simulink model "XWing"  (R2018a)
settings: Solver=VariableStepAuto  StartTime=0.0  StopTime=10.0  RelTol=1e-5  AbsTol=1e-5
PostLoadFcn:
  | Lcm = 3.2;
undefined symbols (not defined in the file): X, Y, Z
libraries: sm_lib x12, nesl_utility x4
settings Model: Creator=tdenery  LastModifiedBy=smirsky

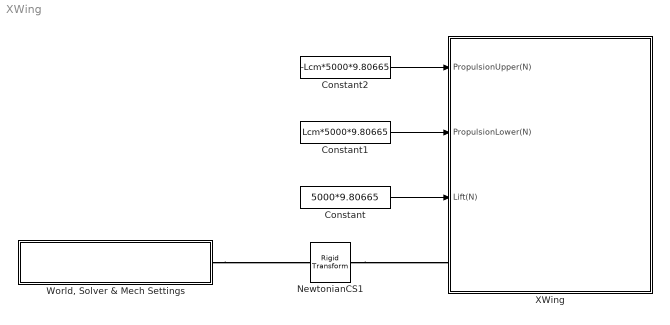
== system XWing ==
  Constant : Constant  Value=5000*9.80665
  Constant1 : Constant  Value=Lcm*5000*9.80665
  Constant2 : Constant  Value=-Lcm*5000*9.80665
  NewtonianCS1 : sm_lib/Frames and Transforms/Rigid Transform  TranslationMethod=Cartesian  TranslationStandardOffset=0  TranslationLengthUnit=m  TranslationStandardAxis=+Z  TranslationCartesianOffset=[0, 0, 0]  TranslationROffset=0  TranslationROffsetUnits=m  TranslationZOffset=0  TranslationZOffsetUnits=m  TranslationThetaOffset=0  TranslationThetaOffsetUnits=deg  RotationMethod=ArbitraryAxis  RotationAngleUnits=deg  RotationStandardAxis=+Z  RotationAngle=0  RotationArbitraryAxis=[1, 0, 0]  FollAlignAxisA=+X  BaseAlignAxisA=+Y  FollAlignAxisB=+Y  BaseAlignAxisB=+Z  RotationSequenceAxes=FollowerAxes  RotationSequence=XYX  RotationSequenceAngles=[0 0 0]  RotationSequenceAnglesUnits=deg  RotationMatrix=[1 0 0; 0 1 0; 0 0 1]
  "World, Solver & Mech Settings" : Subsystem
  XWing : Subsystem  Tag=Force/Torque  mask{PopupParam=Force/Torque}
      mask prompts: PopupParam "Motion Configuration"
      mask TypeOptions PopupParam: Force/Torque | Motion
      mask Callback PopupParam:
      | MechSystem = gcb;
      | MotionConfig = get_param( MechSystem, 'PopupParam' );
      | CurrentConfig = get_param( MechSystem, 'Tag' );
      | if ~strcmp( MotionConfig, CurrentConfig )
      |     MotOutports = find_system(MechSystem,'LookUnderMasks','all','Tag','MechSystemMotorOutport');
      |     ActOutports = find_system(MechSystem,'LookUnderMasks','all','Tag','MechSystemActuatorOutport');
      |     APOutports = find_system(MechSystem,'LookUnderMasks','all','Tag','MechSystemAPOutport');
      |     NMotors = length( MotOutports );
      |     NActuators = length( ActOutports );
      |     NActuatedPrismatics = length( APOutports );
      |     if NMotors > 0
      |         hMotOutports( NMotors ) = 0;
      |         hMotors( NMotors ) = 0;
      |         hMotInports( NMotors ) = 0;
      |         MotNameRoot{NMotors} = '';
      |     end
      |     if NActuators > 0
      |         hActOutports( NActuators ) = 0;
      |         hActuators( NActuators ) = 0;
      |         hActInports( NActuators ) = 0;
      |         ActNameRoot{NActuators} = '';
      |     end
      |     if NActuatedPrismatics > 0
      |         hAPOutports( NActuatedPrismatics ) = 0;
      |         hActuatedPrismatics( NActuatedPrismatics ) = 0;
      |         hAPInports( NActuatedPrismatics ) = 0;
      |         APNameRoot{NActuatedPrismatics} = '';
      |     end
      | 
      |     for i = 1:NMotors
      |         hMotOutports(i) = getSimulinkBlockHandle( MotOutports(i) );
      |         OutportName = get_param( hMotOutports(i), 'Name' );
      |         NameLength = length( OutportName );
      |         MotNameRoot{i} = OutportName( 1:NameLength-2 );
      |         hP = get_param( hMotOutports(i), 'PortHandles' );
      |         hL = get_param( hP.Inport, 'Line' );
      |         hMotors(i) = get_param( hL, 'SrcBlockHandle' );
      |         hpMotor(i) = get_param( hMotors(i), 'PortHandles' );
      |     end
      |     for i = 1:NActuators
      |         hActOutports(i) = getSimulinkBlockHandle( ActOutports(i) );
      |         OutportName = get_param( hActOutports(i), 'Name' );
      |         NameLength = length( OutportName );
      |         ActNameRoot{i} = OutportName( 1:NameLength-2 );
      |         hP = get_param( hActOutports(i), 'PortHandles' );
      |         hL = get_param( hP.Inport, 'Line' );
      |         hActuators(i) = get_param( hL, 'SrcBlockHandle' );
      |         hpActuator(i) = get_param( hActuators(i), 'PortHandles' );
      |     end
      |     for i = 1:NActuatedPrismatics
      |         hAPOutports(i) = getSimulinkBlockHandle( APOutports(i) );
      |         OutportName = get_param( hAPOutports(i), 'Name' );
      |         NameLength = length( OutportName );
      |         APNameRoot{i} = OutportName( 1:NameLength-2 );
      |         hP = get_param( hAPOutports(i), 'PortHandles' );
      |         hL = get_param( hP.Inport, 'Line' );
      |         hActuatedPrismatics(i) = get_param( hL, 'SrcBlockHandle' );
      |         hpActuatedPrismatic(i) = get_param( hActuatedPrismatics(i), 'PortHandles' );
      |     end
      | 
      |     if strcmp( MotionConfig, 'Force/Torque' ) || strcmp( MotionConfig, 'Motion' )
      | 
      |         for i = 1:NMotors
      |             if isempty( hpMotor(i).Inport )
      |                 hMotInports(i) = add_block( 'simulink/Sources/In1', [MechSystem, '/Fred', num2str(i)] );
      |                 OutPos = get_param( MotOutports(i), 'Position' );
      |                 InPos = OutPos{1} + [-300, 0, -300, 0];
      |                 set_param( hMotInports(i), 'Position', ['[', num2str(InPos(1)), ',', num2str(InPos(2)), ',', num2str(InPos(3)), ',', num2str(InPos(4)), ']'] );
      |                 set_param( hMotInports(i), 'Tag', 'MechSystemMotorInport' );
      |             else
      |                 hP = hpMotor(i).Inport;
      |                 hL = get_param( hP, 'Line' );
      |                 hMotInports(i) = get_param( hL, 'SrcBlockHandle' );
      |             end
      |         end
      |         for i = 1:NActuators
      |             if isempty( hpActuator(i).Inport )
      |                 hActInports(i) = add_block( 'simulink/Sources/In1', [MechSystem, '/Fred', num2str(i)] );
      |                 OutPos = get_param( ActOutports(i), 'Position' );
      |                 InPos = OutPos{1} + [-300, 0, -300, 0];
      |                 set_param( hActInports(i), 'Position', ['[', num2str(InPos(1)), ',', num2str(InPos(2)), ',', num2str(InPos(3)), ',', num2str(InPos(4)), ']'] );
      |                 set_param( hActInports(i), 'Tag', 'MechSystemACtuatorInport' );
      |             else
      |                 hP = hpActuator(i).Inport;
      |                 hL = get_param( hP, 'Line' );
      |                 hActInports(i) = get_param( hL, 'SrcBlockHandle' );
      |             end
      |         end
      |         for i = 1:NActuatedPrismatics
      |             if isempty( hpActuatedPrismatic(i).Inport )
      |                 hAPInports(i) = add_block( 'simulink/Sources/In1', [MechSystem, '/Fred', num2str(i)] );
      |                 OutPos = get_param( APOutports(i), 'Position' );
      |                 InPos = OutPos{1} + [-300, 0, -300, 0];
      |                 set_param( hAPInports(i), 'Position', ['[', num2str(InPos(1)), ',', num2str(InPos(2)), ',', num2str(InPos(3)), ',', num2str(InPos(4)), ']'] );
      |                 set_param( hAPInports(i), 'Tag', 'MechSystemACtuatorInport' );
      |             else
      |                 hP = hpActuatedPrismatic(i).Inport;
      |                 hL = get_param( hP, 'Line' );
      |                 hAPInports(i) = get_param( hL, 'SrcBlockHandle' );
      |             end
      |         end
      | 
      |         if strcmp( MotionConfig, 'Force/Torque' )
      |             set_param( MechSystem, 'Tag', 'Force/Torque' );
      |             for i = 1:NMotors
      |                 o = get_param( hMotors(i), 'Object' );
      |                 o.MotorType = 'Torque';
      |                 set_param( hMotInports(i), 'Name', [MotNameRoot{i}, '(N*m)'] );
      |                 hP = get_param( hMotInports(i), 'PortHandles' );
      |                 hL = get_param( hP.Outport, 'Line' );
      |                 if hL ~= -1
      |                     delete_line( hL );
      |                 end
      |                 add_line( MechSystem, [get_param( hMotInports(i), 'Name' ), '/1'], [get_param( hMotors(i), 'Name' ), '/1'] );
      |             end
      |             for i = 1:NActuators
      |                 o = get_param( hActuators(i), 'Object' );
      |                 o.ActuationType = 'Force';
      |                 set_param( hActInports(i), 'Name', [ActNameRoot{i}, '(N)'] );
      |                 hP = get_param( hActInports(i), 'PortHandles' );
      |                 hL = get_param( hP.Outport, 'Line' );
      |                 if hL ~= -1
      |                     delete_line( hL );
      |                 end
      |                 add_line( MechSystem, [get_param( hActInports(i), 'Name' ), '/1'], [get_param( hActuators(i), 'Name' ), '/1'] );
      |             end
      |             for i = 1:NActuatedPrismatics
      |                 o = get_param( hActuatedPrismatics(i), 'Object' );
      |                 o.ActuationType = 'Force';
      |                 set_param( hAPInports(i), 'Name', [APNameRoot{i}, '(N)'] );
      |                 hP = get_param( hAPInports(i), 'PortHandles' );
      |                 hL = get_param( hP.Outport, 'Line' );
      |                 if hL ~= -1
      |                     delete_line( hL );
      |                 end
      |                 add_line( MechSystem, [get_param( hAPInports(i), 'Name' ), '/1'], [get_param( hActuatedPrismatics(i), 'Name' ), '/1'] );
      |             end
      |        elseif strcmp( MotionConfig, 'Motion' )
      |             set_param( MechSystem, 'Tag', 'Motion' );
      |             for i = 1:NMotors
      |                 o = get_param( hMotors(i), 'Object' );
      |                 o.MotorType = 'Motion';
      |                 set_param( hMotInports(i), 'Name', [MotNameRoot{i}, '_pva'] );
      |                 hP = get_param( hMotInports(i), 'PortHandles' );
      |                 hL = get_param( hP.Outport, 'Line' );
      |                 if hL ~= -1
      |                     delete_line( hL );
      |                 end
      |                 add_line( MechSystem, [get_param( hMotInports(i), 'Name' ), '/1'], [get_param( hMotors(i), 'Name' ), '/1'] );
      |             end
      |             for i = 1:NActuators
      |                 o = get_param( hActuators(i), 'Object' );
      |                 o.ActuationType = 'Motion';
      |                 set_param( hActInports(i), 'Name', [ActNameRoot{i}, '_pva'] );
      |                 hP = get_param( hActInports(i), 'PortHandles' );
      |                 hL = get_param( hP.Outport, 'Line' );
      |                 if hL ~= -1
      |                     delete_line( hL );
      |                 end
      |                 add_line( MechSystem, [get_param( hActInports(i), 'Name' ), '/1'], [get_param( hActuators(i), 'Name' ), '/1'] );
      |             end
      |             for i = 1:NActuatedPrismatics
      |                 o = get_param( hActuatedPrismatics(i), 'Object' );
      |                 o.ActuationType = 'Motion';
      |                 set_param( hAPInports(i), 'Name', [APNameRoot{i}, '_pva'] );
      |                 hP = get_param( hAPInports(i), 'PortHandles' );
      |                 hL = get_param( hP.Outport, 'Line' );
      |                 if hL ~= -1
      |                     delete_line( hL );
      |                 end
      |                 add_line( MechSystem, [get_param( hAPInports(i), 'Name' ), '/1'], [get_param( hActuatedPrismatics(i), 'Name' ), '/1'] );
      |             end
      |         end
      |     elseif strcmp( MotionConfig, 'Inverse' )
      |        set_param( MechSystem, 'Tag', 'Inverse' );
      |        Inports = find_system(MechSystem,'LookUnderMasks','all','Tag','MechSystemMotorInport');
      |        for i = 1:NMotors
      |             hP = get_param( Inports{i}, 'PortHandles' );
      |             hL = get_param( hP.Outport, 'Line' );
      |             delete_line( hL );
      |             delete_block( Inports{i} );
      |             o = get_param( hMotors(i), 'Object' );
      |             o.MotorType = 'Inverse';
      |        end
      |        Inports = find_system(MechSystem,'LookUnderMasks','all','Tag','MechSystemActuatorInport');
      |        for i = 1:NActuators
      |             hP = get_param( Inports{i}, 'PortHandles' );
      |             hL = get_param( hP.Outport, 'Line' );
      |             delete_line( hL );
      |             delete_block( Inports{i} );
      |             o = get_param( hActuators(i), 'Object' );
      |             o.ActuatorType = 'Inverse';
      |        end
      |        Inports = find_system(MechSystem,'LookUnderMasks','all','Tag','MechSystemAPInport');
      |        for i = 1:NActuatedPrismatics
      |             hP = get_param( Inports{i}, 'PortHandles' );
      |             hL = get_param( hP.Outport, 'Line' );
      |             delete_line( hL );
      |             delete_block( Inports{i} );
      |             o = get_param( hActuatedPrismatics(i), 'Object' );
      |             o.ActuatorType = 'Inverse';
      |        end
      |     end
      | end
      | clear( 'hMechSystem', 'hOutports', 'i', 'InportName', 'Inports', 'MotionConfig', 'Motors', 'NameLength', 'NameRoot', 'NMotors', 'Outports', 'hInports', 'hL', 'hMotors', 'hP', 'hpMotor', 'InPos', 'MechSystem', 'o', 'OutportName', 'OutPos', 'ActOutports', 'hMotInports', 'hMotOutports', 'MotNameRoot', 'MotOutports', 'NActuators', 'ActNameRoot', 'hActInports', 'hActOutports', 'hActuators', 'hpActuator', 'hpPrisJoint', 'hPrisJoint', 'PrisJointLC2Pos', 'APNameRoot', 'APOutports', 'hActuatedPrismatics', 'hAPInports', 'hAPOutports', 'hpActuatedPrismatic', 'NActuatedPrismatics' );
  wires:
  Constant/1 -> XWing/3(Lift(N))
  Constant1/1 -> XWing/2(PropulsionLower(N))
  Constant2/1 -> XWing/1(PropulsionUpper(N))
  connections:
  "World, Solver & Mech Settings"/RConn1 -- NewtonianCS1/LConn1
  NewtonianCS1/RConn1 -- XWing/LConn1

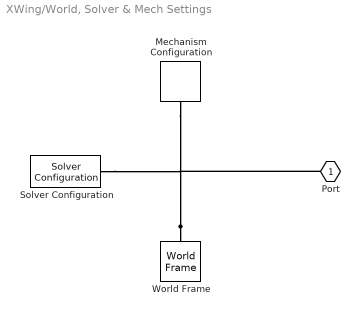
== system XWing/World, Solver & Mech Settings ==
  Mechanism Configuration : sm_lib/Utilities/Mechanism Configuration  UniformGravity=Constant  GravityVector=[0 0 -9.80665]  GravityUnits=m/s^2  LinearizationDelta=0.001
  Solver Configuration : nesl_utility/Solver Configuration  PhysicalDomain=network_engine_domain  SubClassName=solver  LeftPortType=input  RightPortType=generic  Tones=[]  Harmonics=[]  SimulateNoise=off  Profile=off  UseLocalSampling=off  EnableSwitchedLinearOptims=on  FrequencyDomain=off  UseCCode=off  RelTol=0.001  AbsTol=1e-06  MinStep=1e-09  ToWorkspace=off  RevertToSquareIcSolve=off  NumHomotopyIterations=100  PhasorMode=off  PhasorModeNumHarmonics=1  DoDC=off  ResidualTolerance=1e-05  UseLocalSolver=off  LocalSolverChoice=NE_BACKWARD_EULER_ADVANCER  LocalSolverSampleTime=0.001  DoFixedCost=off  MaxNonlinIter=3  MaxModeIter=2  LinearAlgebra=Sparse  EquationFormulation=NE_TIME_EF  DelaysMemoryBudget=1024  AutomaticFiltering=on  FilteringTimeConstant=0.001
  World Frame : sm_lib/Frames and Transforms/World Frame
  Port : PMIOPort  Side=Right
  connections:
  World Frame/RConn1 -- Solver Configuration/RConn1 -- Mechanism Configuration/RConn1 -- Port/RConn1

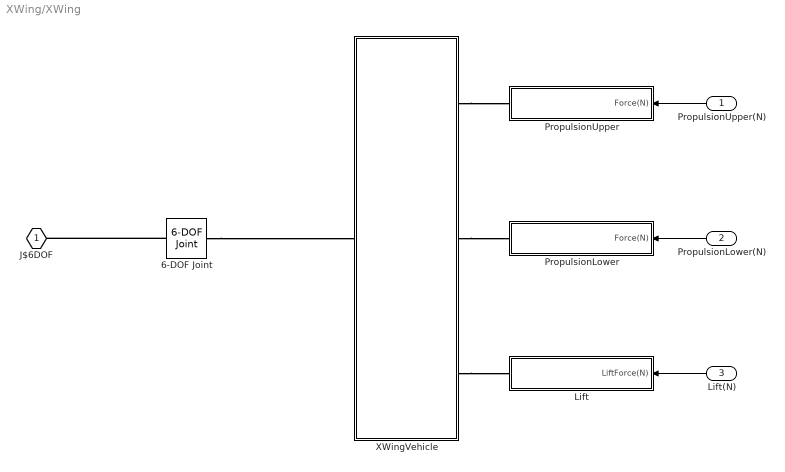
== system XWing/XWing ==
  PropulsionUpper(N) : Inport
  PropulsionLower(N) : Inport  Port=2
  Lift(N) : Inport  Port=3
  6-DOF Joint : sm_lib/Joints/6-DOF Joint  SenseConstraintForce=off  SenseConstraintForceX=off  SenseConstraintForceY=off  SenseConstraintForceZ=off  SenseConstraintTorque=off  SenseConstraintTorqueX=off  SenseConstraintTorqueY=off  SenseConstraintTorqueZ=off  SenseTotalForce=off  SenseTotalForceX=off  SenseTotalForceY=off  SenseTotalForceZ=off  SenseTotalTorque=off  SenseTotalTorqueX=off  SenseTotalTorqueY=off  SenseTotalTorqueZ=off  CompositeWrenchDir=FollowerOnBase  CompositeWrenchFrame=BaseFrame  PxEquilibriumPosition=0  PxEquilibriumPositionUnits=m  PxSpringStiffness=0  PxSpringStiffnessUnits=N/m  PxDampingCoefficient=0  PxDampingCoefficientUnits=N/(m/s)  PxTorqueActuationMode=NoTorque  PxMotionActuationMode=ComputedMotion  PxSensePosition=off  PxSenseVelocity=off  PxSenseAcceleration=off  PxSenseTorqueForce=off  PxPositionTargetSpecify=off  PxPositionTargetPriority=High  PxPositionTargetValue=0  PxPositionTargetValueUnits=m  PxVelocityTargetSpecify=off  PxVelocityTargetPriority=High  PxVelocityTargetValue=0  PxVelocityTargetValueUnits=m/s  PyEquilibriumPosition=0  PyEquilibriumPositionUnits=m  PySpringStiffness=0  PySpringStiffnessUnits=N/m  PyDampingCoefficient=0  PyDampingCoefficientUnits=N/(m/s)  PyTorqueActuationMode=NoTorque  PyMotionActuationMode=ComputedMotion  PySensePosition=off  PySenseVelocity=off  PySenseAcceleration=off  PySenseTorqueForce=off  PyPositionTargetSpecify=off  PyPositionTargetPriority=High  PyPositionTargetValue=0  PyPositionTargetValueUnits=m  PyVelocityTargetSpecify=off  PyVelocityTargetPriority=High  PyVelocityTargetValue=0  PyVelocityTargetValueUnits=m/s  PzEquilibriumPosition=0  PzEquilibriumPositionUnits=m  PzSpringStiffness=0  PzSpringStiffnessUnits=N/m  PzDampingCoefficient=0  PzDampingCoefficientUnits=N/(m/s)  PzTorqueActuationMode=NoTorque  PzMotionActuationMode=ComputedMotion  PzSensePosition=off  PzSenseVelocity=off  PzSenseAcceleration=off  PzSenseTorqueForce=off  PzPositionTargetSpecify=off  PzPositionTargetPriority=High  PzPositionTargetValue=0  PzPositionTargetValueUnits=m  PzVelocityTargetSpecify=off  PzVelocityTargetPriority=High  PzVelocityTargetValue=0  PzVelocityTargetValueUnits=m/s  SphDefPosRotationMethod=None  SphDefPosRotationAngleUnits=deg  SphDefPosRotationStandardAxis=+Z  SphDefPosRotationAngle=0.0  SphDefPosRotationArbitraryAxis=[0 0 1]  SphDefPosFollAlignAxisA=+X  SphDefPosBaseAlignAxisA=+Y  SphDefPosFollAlignAxisB=+Y  SphDefPosBaseAlignAxisB=+Z  SphDefPosRotationSequenceAxes=FollowerAxes  SphDefPosRotationSequence=XYX  SphDefPosRotationSequenceAngles=[0 0 0]  SphDefPosRotationSequenceAnglesUnits=deg  SphDefPosRotationMatrix=[1 0 0; 0 1 0; 0 0 1]  SphEqPosRotationMethod=None  SphEqPosRotationAngleUnits=deg  SphEqPosRotationStandardAxis=+Z  SphEqPosRotationAngle=0.0  SphEqPosRotationArbitraryAxis=[0 0 1]  SphEqPosFollAlignAxisA=+X  SphEqPosBaseAlignAxisA=+Y  SphEqPosFollAlignAxisB=+Y  SphEqPosBaseAlignAxisB=+Z  SphEqPosRotationSequenceAxes=FollowerAxes  SphEqPosRotationSequence=XYX  SphEqPosRotationSequenceAngles=[0 0 0]  SphEqPosRotationSequenceAnglesUnits=deg  SphEqPosRotationMatrix=[1 0 0; 0 1 0; 0 0 1]  SphSpringStiffness=0  SphSpringStiffnessUnits=N*m/deg  SphDampingCoefficient=0  SphDampingCoefficientUnits=N*m/(deg/s)  SphActuateTorqueX=off  SphActuateTorqueY=off  SphActuateTorqueZ=off  SphActuateTorque=off  SphTorqueActuationMode=NoTorque  SphMotionActuationMode=ComputedMotion  SphActuationFrame=BaseFrame  SphSensePosition=off  SphSenseVelocityX=off  SphSenseVelocityY=off  SphSenseVelocityZ=off  SphSenseVelocity=off  SphSenseAccelerationX=off  SphSenseAccelerationY=off  SphSenseAccelerationZ=off  SphSenseAcceleration=off  SphSenseTorqueX=off  SphSenseTorqueY=off  SphSenseTorqueZ=off  SphSenseTorqueForce=off  SphSensingFrame=BaseFrame  SphPositionTargetRotationMethod=None  SphPositionTargetRotationAngleUnits=deg  SphPositionTargetRotationStandardAxis=+Z  SphPositionTargetRotationAngle=0.0  SphPositionTargetRotationArbitraryAxis=[0 0 1]  SphPositionTargetFollAlignAxisA=+X  SphPositionTargetBaseAlignAxisA=+Y  SphPositionTargetFollAlignAxisB=+Y  SphPositionTargetBaseAlignAxisB=+Z  SphPositionTargetRotationSequenceAxes=FollowerAxes  SphPositionTargetRotationSequence=XYX  SphPositionTargetRotationSequenceAngles=[0 0 0]  SphPositionTargetRotationSequenceAnglesUnits=deg  SphPositionTargetRotationMatrix=[1 0 0; 0 1 0; 0 0 1]  SphPositionTargetSpecify=off  SphPositionTargetPriority=High  SphVelocityTargetValue=[0 0 0]  SphVelocityTargetValueUnits=deg/s  SphVelocityTargetSpecify=off  SphVelocityTargetPriority=High  SphVelocityTargetInFollowerFrame=on
  Lift : Subsystem  mask(Applied Force){}
      mask help:
      | Receives a scalar signal that describes force in the local coordinate system for the force, in the z-direction.
      |
      | The units for force are Newtons.
  PropulsionLower : Subsystem  mask(Applied Force){}
      mask help:
      | Receives a scalar signal that describes force in the local coordinate system for the force, in the z-direction.
      |
      | The units for force are Newtons.
  PropulsionUpper : Subsystem  mask(Applied Force){}
      mask help:
      | Receives a scalar signal that describes force in the local coordinate system for the force, in the z-direction.
      |
      | The units for force are Newtons.
  XWingVehicle : Subsystem
  J$6DOF : PMIOPort  Side=Left
  wires:
  PropulsionUpper(N)/1 -> PropulsionUpper/1(Force(N))
  PropulsionLower(N)/1 -> PropulsionLower/1(Force(N))
  Lift(N)/1 -> Lift/1(LiftForce(N))
  connections:
  6-DOF Joint/LConn1 -- J$6DOF/RConn1
  6-DOF Joint/RConn1 -- XWingVehicle/LConn1
  XWingVehicle/RConn1 -- PropulsionUpper/RConn1
  XWingVehicle/RConn2 -- PropulsionLower/RConn1
  XWingVehicle/RConn3 -- Lift/RConn1

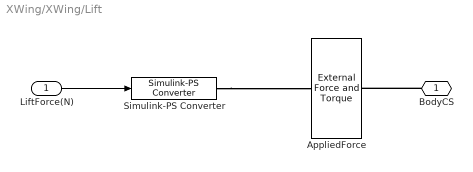
== system XWing/XWing/Lift ==
  LiftForce(N) : Inport
  AppliedForce : sm_lib/Forces and Torques/External Force and Torque  ForceResolutionFrame=AttachedFrame  EnableForceX=off  EnableForceY=off  EnableForceZ=on  EnableForce=off  TorqueResolutionFrame=AttachedFrame  EnableTorqueX=off  EnableTorqueY=off  EnableTorqueZ=off  EnableTorque=off
  Simulink-PS Converter : nesl_utility/Simulink-PS Converter  PhysicalDomain=network_engine_domain  SubClassName=ps_input  LeftPortType=input  RightPortType=output  PseudoPeriodic=off  Frequencies=[]  NoiseDistribution=none  NoiseParameters=[]  Unit=1  AffineConversion=off  FilteringAndDerivatives=zero  SimscapeFilterOrder=1  InputFilterTimeConstant=0.001  UdotUserProvided=1
  BodyCS : PMIOPort  Side=Right
  wires:
  LiftForce(N)/1 -> Simulink-PS Converter/1
  connections:
  Simulink-PS Converter/RConn1 -- AppliedForce/LConn1
  BodyCS/RConn1 -- AppliedForce/RConn1

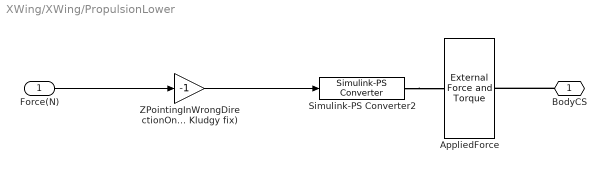
== system XWing/XWing/PropulsionLower ==
  Force(N) : Inport
  AppliedForce : sm_lib/Forces and Torques/External Force and Torque  ForceResolutionFrame=AttachedFrame  EnableForceX=off  EnableForceY=off  EnableForceZ=on  EnableForce=off  TorqueResolutionFrame=AttachedFrame  EnableTorqueX=off  EnableTorqueY=off  EnableTorqueZ=off  EnableTorque=off
  Simulink-PS Converter2 : nesl_utility/Simulink-PS Converter  PhysicalDomain=network_engine_domain  SubClassName=ps_input  LeftPortType=input  RightPortType=output  PseudoPeriodic=off  Frequencies=[]  NoiseDistribution=none  NoiseParameters=[]  Unit=1  AffineConversion=off  FilteringAndDerivatives=zero  SimscapeFilterOrder=1  InputFilterTimeConstant=0.001  UdotUserProvided=1
  ZPointingInWrongDirectionOnFrame (This is a Kludgy fix) : Gain  Gain=-1
  BodyCS : PMIOPort  Side=Right
  wires:
  Force(N)/1 -> ZPointingInWrongDirectionOnFrame (This is a Kludgy fix)/1
  ZPointingInWrongDirectionOnFrame (This is a Kludgy fix)/1 -> Simulink-PS Converter2/1
  connections:
  BodyCS/RConn1 -- AppliedForce/RConn1
  Simulink-PS Converter2/RConn1 -- AppliedForce/LConn1

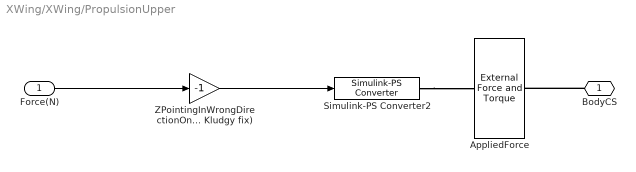
== system XWing/XWing/PropulsionUpper ==
  Force(N) : Inport
  AppliedForce : sm_lib/Forces and Torques/External Force and Torque  ForceResolutionFrame=AttachedFrame  EnableForceX=off  EnableForceY=off  EnableForceZ=on  EnableForce=off  TorqueResolutionFrame=AttachedFrame  EnableTorqueX=off  EnableTorqueY=off  EnableTorqueZ=off  EnableTorque=off
  Simulink-PS Converter2 : nesl_utility/Simulink-PS Converter  PhysicalDomain=network_engine_domain  SubClassName=ps_input  LeftPortType=input  RightPortType=output  PseudoPeriodic=off  Frequencies=[]  NoiseDistribution=none  NoiseParameters=[]  Unit=1  AffineConversion=off  FilteringAndDerivatives=zero  SimscapeFilterOrder=1  InputFilterTimeConstant=0.001  UdotUserProvided=1
  ZPointingInWrongDirectionOnFrame (This is a Kludgy fix) : Gain  Gain=-1
  BodyCS : PMIOPort  Side=Right
  wires:
  Force(N)/1 -> ZPointingInWrongDirectionOnFrame (This is a Kludgy fix)/1
  ZPointingInWrongDirectionOnFrame (This is a Kludgy fix)/1 -> Simulink-PS Converter2/1
  connections:
  BodyCS/RConn1 -- AppliedForce/RConn1
  Simulink-PS Converter2/RConn1 -- AppliedForce/LConn1

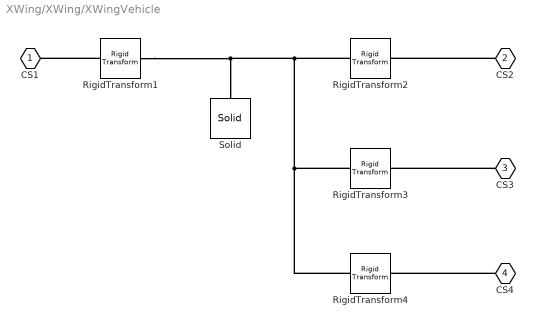
== system XWing/XWing/XWingVehicle ==
  RigidTransform1 : sm_lib/Frames and Transforms/Rigid Transform  TranslationMethod=Cartesian  TranslationStandardOffset=0  TranslationLengthUnit=m  TranslationStandardAxis=+Z  TranslationCartesianOffset=[2.5215971710939309, 3.2616068986551572E-06, 2.4152810404276371E-06]  TranslationROffset=0  TranslationROffsetUnits=m  TranslationZOffset=0  TranslationZOffsetUnits=m  TranslationThetaOffset=0  TranslationThetaOffsetUnits=deg  RotationMethod=ArbitraryAxis  RotationAngleUnits=deg  RotationStandardAxis=+Z  RotationAngle=15.00000000000002  RotationArbitraryAxis=[-0.99999999999999845, 0, 0]  FollAlignAxisA=+X  BaseAlignAxisA=+Y  FollAlignAxisB=+Y  BaseAlignAxisB=+Z  RotationSequenceAxes=FollowerAxes  RotationSequence=XYX  RotationSequenceAngles=[0 0 0]  RotationSequenceAnglesUnits=deg  RotationMatrix=[1 0 0; 0 1 0; 0 0 1]
  RigidTransform2 : sm_lib/Frames and Transforms/Rigid Transform  TranslationMethod=Cartesian  TranslationStandardOffset=0  TranslationLengthUnit=m  TranslationStandardAxis=+Z  TranslationCartesianOffset=[-2.5215971710939309, -0.097059667263051347, 0.36221900771008292]  TranslationROffset=0  TranslationROffsetUnits=m  TranslationZOffset=0  TranslationZOffsetUnits=m  TranslationThetaOffset=0  TranslationThetaOffsetUnits=deg  RotationMethod=ArbitraryAxis  RotationAngleUnits=deg  RotationStandardAxis=+Z  RotationAngle=269.02379959839919  RotationArbitraryAxis=[-0.1294283079955636, 0.98310560276035985, 0.1294283079955636]  FollAlignAxisA=+X  BaseAlignAxisA=+Y  FollAlignAxisB=+Y  BaseAlignAxisB=+Z  RotationSequenceAxes=FollowerAxes  RotationSequence=XYX  RotationSequenceAngles=[0 0 0]  RotationSequenceAnglesUnits=deg  RotationMatrix=[1 0 0; 0 1 0; 0 0 1]
  RigidTransform3 : sm_lib/Frames and Transforms/Rigid Transform  TranslationMethod=Cartesian  TranslationStandardOffset=0  TranslationLengthUnit=m  TranslationStandardAxis=+Z  TranslationCartesianOffset=[-2.5215971710939309, 0.097054616563839194, -0.36222536200671829]  TranslationROffset=0  TranslationROffsetUnits=m  TranslationZOffset=0  TranslationZOffsetUnits=m  TranslationThetaOffset=0  TranslationThetaOffsetUnits=deg  RotationMethod=ArbitraryAxis  RotationAngleUnits=deg  RotationStandardAxis=+Z  RotationAngle=269.02379959839919  RotationArbitraryAxis=[-0.1294283079955636, 0.98310560276035985, 0.1294283079955636]  FollAlignAxisA=+X  BaseAlignAxisA=+Y  FollAlignAxisB=+Y  BaseAlignAxisB=+Z  RotationSequenceAxes=FollowerAxes  RotationSequence=XYX  RotationSequenceAngles=[0 0 0]  RotationSequenceAnglesUnits=deg  RotationMatrix=[1 0 0; 0 1 0; 0 0 1]
  RigidTransform4 : sm_lib/Frames and Transforms/Rigid Transform  TranslationMethod=Cartesian  TranslationStandardOffset=0  TranslationLengthUnit=m  TranslationStandardAxis=+Z  TranslationCartesianOffset=[-2.5215971710939309, -2.5253496060759038E-06, -3.1771483177051082E-06]  TranslationROffset=0  TranslationROffsetUnits=m  TranslationZOffset=0  TranslationZOffsetUnits=m  TranslationThetaOffset=0  TranslationThetaOffsetUnits=deg  RotationMethod=ArbitraryAxis  RotationAngleUnits=deg  RotationStandardAxis=+Z  RotationAngle=15.00000000000002  RotationArbitraryAxis=[0.99999999999999845, 0, 0]  FollAlignAxisA=+X  BaseAlignAxisA=+Y  FollAlignAxisB=+Y  BaseAlignAxisB=+Z  RotationSequenceAxes=FollowerAxes  RotationSequence=XYX  RotationSequenceAngles=[0 0 0]  RotationSequenceAnglesUnits=deg  RotationMatrix=[1 0 0; 0 1 0; 0 0 1]
  Solid : sm_lib/Body Elements/Solid  InertiaType=Custom  Mass=5000  MassUnits=kg  CenterOfMass=[0 0 0]  CenterOfMassUnits=m  MomentsOfInertia=[6054.0639566245882, 18392.66271822443, 22548.802163355522]  MomentsOfInertiaUnits=kg*m^2  ProductsOfInertia=[-1199.74045372458, -0.031428433661443239, -0.024980934207831079]  ProductsOfInertiaUnits=kg*m^2  DensityBased=on  Density=1000  DensityUnits=kg/(m^3)  DoExposeReferenceFrame=on  SerializedFrames=<Frames/>  GraphicType=FromGeometry  MarkerShape=Sphere  MarkerSize=10  MarkerSizeUnits=m  GraphicVisPropType=SimpleVisualProperties  GraphicDiffuseColor=[0.203922; 0.501961; 0.501961]  GraphicSpecularColor=[0.203922; 0.501961; 0.501961]  GraphicAmbientColor=[0.203922; 0.501961; 0.501961]  GraphicEmissiveColor=[0.203922; 0.501961; 0.501961]  GraphicShininess=75  GraphicOpacity=1.0  GeometryShape=FromFile  RectangleSize=[1 1]  RectangleSizeUnits=m  BrickDimensions=[1 1 1]  BrickDimensionUnits=m  CylinderRadius=1  CylinderRadiusUnits=m  CylinderLength=1  CylinderLengthUnits=m  SphereRadius=1  SphereRadiusUnits=m  EllipsoidRadii=[1 1 1]  EllipsoidRadiiUnits=m  ExtrusionCrossSection=[1 1; -1 1; -1 -1; 1 -1]  ExtrusionCrossSectionUnits=m  ExtrusionLength=1  ExtrusionLengthUnits=m  PolygonNumSides=3  PolygonOuterRadius=1  PolygonOuterRadiusUnits=m  ExtGeomFileType=STL  ExtGeomFileName=XWingVehicle_1.stl  ExtGeomFileUnits=m  RevolutionCrossSection=[1 1; 1 -1; 2 -1; 2 1]  RevolutionCrossSectionUnits=m  RevolutionExtent=Full  RevolutionAngle=180  RevolutionAngleUnits=deg
  "CS1 " : PMIOPort  Side=Left
  CS2 : PMIOPort  Port=2  Side=Right
  CS3 : PMIOPort  Port=3  Side=Right
  CS4 : PMIOPort  Port=4  Side=Right
  connections:
  RigidTransform1/LConn1 -- "CS1 "/RConn1
  RigidTransform3/LConn1 -- Solid/RConn1 -- RigidTransform1/RConn1 -- RigidTransform2/LConn1 -- RigidTransform4/LConn1
  CS2/RConn1 -- RigidTransform2/RConn1
  CS3/RConn1 -- RigidTransform3/RConn1
  CS4/RConn1 -- RigidTransform4/RConn1
